simulink model "multiCopter"  (R2014a)
settings: Solver=FixedStepDiscrete  StartTime=0.0  StopTime=simTime  FixedStep=controlDT  RelTol=1e-3
values from neighbouring files (symbols this model uses):
  controlDT = 1 / 500    (= 0.002)    [setup.m]
  filterDT = 1 / 100    (= 0.01)    [setup.m]
settings Model: Creator=John Ihlein  LastModifiedBy=John Ihlein
settings DataIOCC: SaveFormat=Structure
settings OptimizationCC: InlineParams=on  DefaultUnderspecifiedDataType=single  InlineInvariantSignals=on  PassReuseOutputArgsAs=Individual arguments  StateBitsets=on  DataBitsets=on  ZeroExternalMemoryAtStartup=off  ZeroInternalMemoryAtStartup=off  EfficientFloat2IntCast=on  OptimizeModelRefInitCode=on  LifeSpan=1
settings DebuggingCC: ParameterPrecisionLossMsg=none  UniqueDataStoreMsg=error  AssertControl=DisableAll
settings HardwareCC: ProdLargestAtomicInteger=Integer  ProdLargestAtomicFloat=Float  ProdIntDivRoundTo=Zero  ProdEndianess=LittleEndian  ProdHWDeviceType=STMicroelectronics->STM32F4xx 32-bit Cortex-M4
settings RTWCC: SystemTargetFile=ert.tlc  GenCodeOnly=on  TemplateMakefile=ert_default_tmf  Description=Embedded Coder  ProcessScript=ert_make_rtw_hook
settings CodeAppCC: IgnoreCustomStorageClasses=off  IgnoreTestpoints=on
settings ERTTargetCC: ParMdlRefBuildCompliant=on  CompOptLevelCompliant=on  ConcurrentExecutionCompliant=on  IncludeMdlTerminateFcn=off  ERTFirstTimeCompliant=on  SupportNonFinite=off  ParenthesesLevel=Maximum  ModelStepFunctionPrototypeControlCompliant=on  CPPClassGenCompliant=on  InlinedParameterPlacement=Hierarchical  ERTCustomFileTemplate=example_file_process.tlc  ERTFilePackagingFormat=Compact

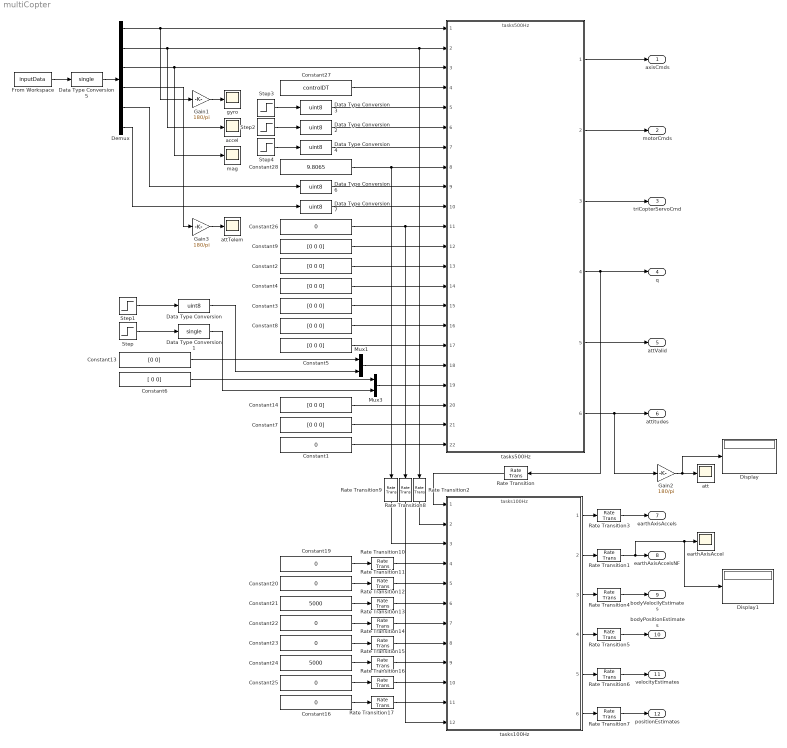
== system multiCopter ==
  Constant1 : Constant  Value=0  OutDataTypeStr=uint8  SampleTime=controlDT
  Constant13 : Constant  Value=[0 0]  OutDataTypeStr=uint8  SampleTime=controlDT
  Constant14 : Constant  Value=[0 0 0]  OutDataTypeStr=uint8  SampleTime=controlDT
  Constant16 : Constant  Value=0  OutDataTypeStr=uint8  SampleTime=filterDT
  Constant{19..20,22..23} (4 alike) : Constant  Value=0  OutDataTypeStr=int32  SampleTime=filterDT
  Constant{2..3,5,7,9} (5 alike) : Constant  Value=[0 0 0]  OutDataTypeStr=single  SampleTime=controlDT
  Constant21 : Constant  Value=5000  OutDataTypeStr=int32  SampleTime=filterDT
  Constant24 : Constant  Value=5000  OutDataTypeStr=int32  SampleTime=filterDT
  Constant25 : Constant  Value=0  OutDataTypeStr=single  SampleTime=filterDT
  Constant26 : Constant  Value=0  OutDataTypeStr=single  SampleTime=controlDT
  Constant27 : Constant  Value=controlDT  OutDataTypeStr=single  SampleTime=controlDT
  Constant28 : Constant  Value=9.8065  OutDataTypeStr=single  SampleTime=controlDT
  Constant4 : Constant  Value=[0 0 0]  OutDataTypeStr=uint8  SampleTime=controlDT
  Constant6 : Constant  Value=[ 0 0]  OutDataTypeStr=single  SampleTime=controlDT
  Constant8 : Constant  Value=[0 0 0]  OutDataTypeStr=uint8  SampleTime=controlDT
  Data Type Conversion{,2..4,6..7} (6 alike) : DataTypeConversion  OutDataTypeStr=uint8
  Data Type Conversion1 : DataTypeConversion  OutDataTypeStr=single
  Data Type Conversion5 : DataTypeConversion  OutDataTypeStr=single
  Demux : Demux  Outputs=[3 3 3 3 1 1]
  Display : Display
  Display1 : Display
  From Workspace : FromWorkspace  VariableName=inputData  SampleTime=controlDT
  Gain1 : Gain  Gain=180/pi
  Gain2 : Gain  Gain=180/pi
  Gain3 : Gain  Gain=180/pi
  Mux1 : Mux  Inputs=[2 1]
  Mux3 : Mux  Inputs=[2 1]
  Rate Transition{,1..17} (18 alike) : RateTransition
  Step : Step  Time=3  Before=2250  SampleTime=controlDT
  Step1 : Step  Time=3  SampleTime=controlDT
  Step2 : Step  Time=3 * controlDT  SampleTime=0
  Step3 : Step  Time=3 * controlDT  SampleTime=0
  Step4 : Step  Time=3 * controlDT  SampleTime=0
  accel : Scope
      settings: SaveName=ScopeData2
  att : Scope
  attTelem : Scope
      settings: SaveName=ScopeData5
  earthAxisAccel : Scope
      settings: SaveName=ScopeData4
  gyro : Scope
  mag : Scope
      settings: SaveName=ScopeData3
  tasks100Hz : ModelReference  ModelNameDialog=tasks100Hz  SimulationMode=Normal  ModelReferenceVersion=1.392  CopyOfModelName=tasks100Hz  DefaultDataLogging=on
  tasks500Hz : ModelReference  ModelNameDialog=tasks500Hz  SimulationMode=Normal  ModelReferenceVersion=1.389  CopyOfModelName=tasks500Hz  DefaultDataLogging=on
  axisCmds : Outport  OutDataTypeStr=single  PortDimensions=4  SampleTime=controlDT
  motorCmds : Outport  Port=2  OutDataTypeStr=single  PortDimensions=numMotors  SampleTime=controlDT
  triCopterServoCmd : Outport  Port=3  OutDataTypeStr=single  PortDimensions=1  SampleTime=controlDT
  q : Outport  Port=4  OutDataTypeStr=single  PortDimensions=4  SampleTime=controlDT
  attValid : Outport  Port=5  OutDataTypeStr=uint8  PortDimensions=1  SampleTime=controlDT
  attitudes : Outport  Port=6  OutDataTypeStr=single  PortDimensions=3  SampleTime=controlDT
  earthAxisAccels : Outport  Port=7
  earthAxisAccelsNF : Outport  Port=8
  bodyVelocilyEstimates : Outport  Port=9
  bodyPositionEstimates : Outport  Port=10
  velocityEstimates : Outport  Port=11
  positionEstimates : Outport  Port=12
  wires:
  Demux/1 -> tasks500Hz/1, Gain1/1
  Demux/3 -> tasks500Hz/3, mag/1
  Demux/6 -> Data Type Conversion7/1
  tasks500Hz/1 -> axisCmds/1
  Constant9/1 -> tasks500Hz/12
  tasks500Hz/6 -> attitudes/1, Gain2/1
  Constant1/1 -> tasks500Hz/22
  Constant2/1 -> tasks500Hz/13
  Constant3/1 -> tasks500Hz/15
  Constant5/1 -> tasks500Hz/17
  Constant7/1 -> tasks500Hz/21
  Constant4/1 -> tasks500Hz/14
  Constant8/1 -> tasks500Hz/16
  Mux1/1 -> tasks500Hz/18
  Constant13/1 -> Mux1/1
  Mux3/1 -> tasks500Hz/19
  Constant6/1 -> Mux3/1
  Step/1 -> Data Type Conversion1/1
  Step1/1 -> Data Type Conversion/1
  Data Type Conversion/1 -> Mux1/2
  Data Type Conversion1/1 -> Mux3/2
  tasks500Hz/2 -> motorCmds/1
  tasks500Hz/3 -> triCopterServoCmd/1
  Rate Transition3/1 -> earthAxisAccels/1
  tasks100Hz/1 -> Rate Transition3/1
  Rate Transition/1 -> tasks100Hz/1
  Rate Transition4/1 -> bodyVelocilyEstimates/1
  Rate Transition5/1 -> bodyPositionEstimates/1
  Rate Transition6/1 -> velocityEstimates/1
  Rate Transition7/1 -> positionEstimates/1
  Constant16/1 -> Rate Transition17/1
  Rate Transition9/1 -> tasks100Hz/3
  Constant19/1 -> Rate Transition10/1
  Constant20/1 -> Rate Transition11/1
  Constant21/1 -> Rate Transition12/1
  Constant25/1 -> Rate Transition16/1
  Constant22/1 -> Rate Transition13/1
  Constant23/1 -> Rate Transition14/1
  Constant24/1 -> Rate Transition15/1
  tasks100Hz/3 -> Rate Transition4/1
  tasks100Hz/6 -> Rate Transition7/1
  tasks100Hz/5 -> Rate Transition6/1
  tasks100Hz/4 -> Rate Transition5/1
  tasks100Hz/2 -> Rate Transition1/1
  Constant26/1 -> tasks500Hz/11, Rate Transition8/1
  tasks500Hz/5 -> attValid/1
  Data Type Conversion4/1 -> tasks500Hz/7
  Step2/1 -> Data Type Conversion2/1
  Step4/1 -> Data Type Conversion4/1
  Step3/1 -> Data Type Conversion3/1
  Constant14/1 -> tasks500Hz/20
  tasks500Hz/4 -> Rate Transition/1, q/1
  Data Type Conversion2/1 -> tasks500Hz/6
  Data Type Conversion3/1 -> tasks500Hz/5
  Constant27/1 -> tasks500Hz/4
  Demux/5 -> Data Type Conversion6/1
  Constant28/1 -> tasks500Hz/8, Rate Transition9/1
  Gain1/1 -> gyro/1
  Data Type Conversion5/1 -> Demux/1
  Gain2/1 -> att/1, Display/1
  Rate Transition1/1 -> Display1/1, earthAxisAccel/1, earthAxisAccelsNF/1
  Rate Transition2/1 -> tasks100Hz/2
  Demux/2 -> tasks500Hz/2, Rate Transition2/1, accel/1
  Rate Transition8/1 -> tasks100Hz/12
  Rate Transition10/1 -> tasks100Hz/4
  Rate Transition11/1 -> tasks100Hz/5
  Rate Transition12/1 -> tasks100Hz/6
  Rate Transition13/1 -> tasks100Hz/7
  Rate Transition14/1 -> tasks100Hz/8
  Rate Transition15/1 -> tasks100Hz/9
  Rate Transition16/1 -> tasks100Hz/10
  Rate Transition17/1 -> tasks100Hz/11
  From Workspace/1 -> Data Type Conversion5/1
  Gain3/1 -> attTelem/1
  Demux/4 -> Gain3/1
  Data Type Conversion6/1 -> tasks500Hz/9
  Data Type Conversion7/1 -> tasks500Hz/10
